simulink model "ME561FinalProjectSimulink_ContinuousNoFbOptimized"  (R2020a)
settings: Solver=ode5  StartTime=0.0  StopTime=800  FixedStep=0.01  RelTol=1e-3
values from neighbouring files (symbols this model uses):
  dB = 0.87    [ME561FinalProject.m]
  g = -9.81    [ME561FinalProject.m]
  JB = 66    [ME561FinalProject.m]
  Kd = 195    [ME561FinalProject.m]
  Ki = 3000    [ME561FinalProject.m]
  Kn = 462    [ME561FinalProject.m]
  Kp = 450    [ME561FinalProject.m]
  maxControlOutput = max(abs(controlOutput))    [ME561FinalProject.m]
  mB = 76    [ME561FinalProject.m]
  thetaRef = 0    [ME561FinalProject.m]
  timeDelay = 0.171    [ME561FinalProject.m]
  timeNoise = 100    [ME561FinalProject.m]
libraries: simulink x1
settings Model: Creator=jcferris  LastModifiedBy=jcferris

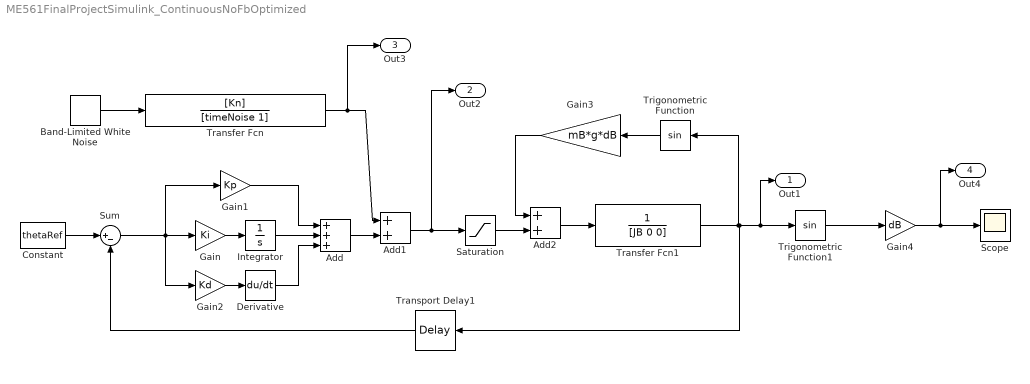
== system ME561FinalProjectSimulink_ContinuousNoFbOptimized ==
  Add : Sum  Inputs=+++
  Add1 : Sum
  Add2 : Sum
  Band-Limited White Noise : simulink/Sources/Band-Limited White Noise  Cov=[0.01]  Ts=0.01  seed=[23341]
  Constant : Constant  Value=thetaRef
  Derivative : Derivative  CoefficientInTFapproximation=0
  Gain : Gain  Gain=Ki
  Gain1 : Gain  Gain=Kp
  Gain2 : Gain  Gain=Kd
  Gain3 : Gain  Gain=mB*g*dB
  Gain4 : Gain  Gain=dB
  Integrator : Integrator
  Saturation : Saturate  UpperLimit=maxControlOutput  LowerLimit=-maxControlOutput
  Scope : Scope
  Sum : Sum  Inputs=|+-
  Transfer Fcn : TransferFcn  Numerator=[Kn]  Denominator=[timeNoise 1]
  Transfer Fcn1 : TransferFcn  Denominator=[JB 0 0]
  Transport Delay1 : TransportDelay  DelayTime=timeDelay
  Trigonometric Function : Trigonometry
  Trigonometric Function1 : Trigonometry
  Out1 : Outport  SignalName=thetaOut
  Out2 : Outport  Port=2  SignalName=controlOutput
  Out3 : Outport  Port=3  SignalName=disturb
  Out4 : Outport  Port=4  SignalName=disp
  wires:
  Gain/1 -> Integrator/1
  Gain2/1 -> Derivative/1
  Sum/1 -> Gain2/1, Gain1/1, Gain/1
  Constant/1 -> Sum/1
  Band-Limited White Noise/1 -> Transfer Fcn/1
  Integrator/1 -> Add/2
  Gain1/1 -> Add/1
  Derivative/1 -> Add/3
  Add/1 -> Add1/2
  Transfer Fcn/1 -> Out3/1, Add1/1
  Add2/1 -> Transfer Fcn1/1
  Transfer Fcn1/1 -> Transport Delay1/1, Trigonometric Function1/1, Out1/1, Trigonometric Function/1
  Trigonometric Function/1 -> Gain3/1
  Gain3/1 -> Add2/1
  Transport Delay1/1 -> Sum/2
  Trigonometric Function1/1 -> Gain4/1
  Gain4/1 -> Out4/1, Scope/1
  Add1/1 -> Out2/1, Saturation/1
  Saturation/1 -> Add2/2
